simulink model "sampleModel1527"  (R2023a)
settings: Solver=VariableStepAuto  StartTime=0.0  StopTime=10.0  RelTol=1e-3
libraries: hdlsllib x3, simulink x3
settings Model: Creator=user1  LastModifiedBy=user1

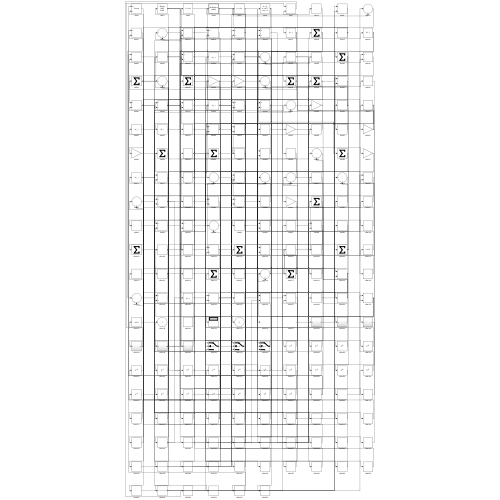
[thumbnail: Simulink's stored preview of the top-level diagram]
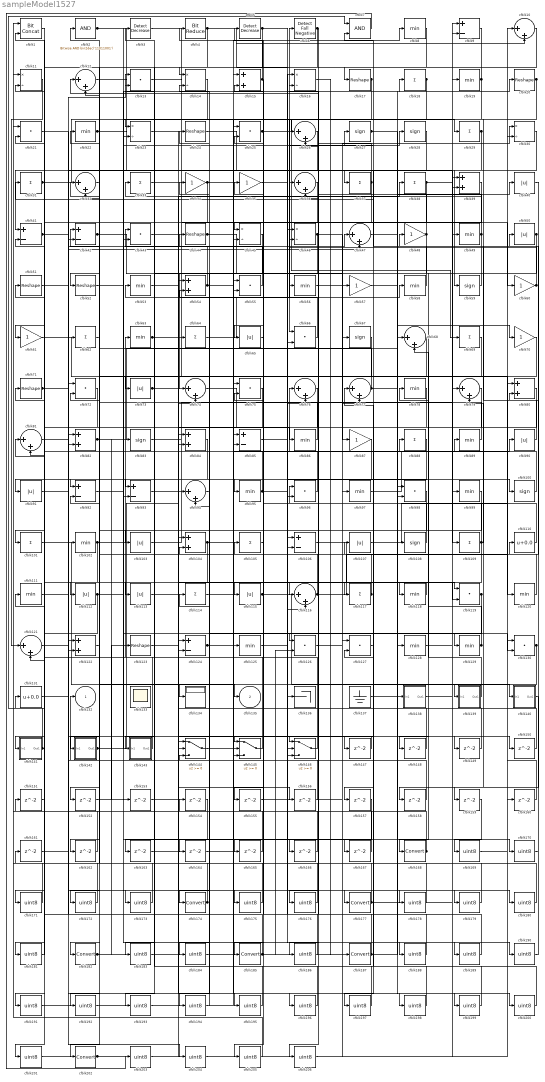
== system sampleModel1527 ==
  cfblk1 : hdlsllib/Logic and Bit Operations/Bit Concat  numInputs=2
  cfblk{10,12,26,32,36,47,68,74,76..77,79,81,94,116,121} (15 alike) : Sum  Inputs=|++
  cfblk{27..28,59,67,83,100,108} (7 alike) : Signum
  cfblk{18,29,31,33,37..38,62,64,69,88,101,105,109,114,117} (15 alike) : Sum  Inputs=+
  cfblk{8,19,22,49,53,56,58,63,78,86,89,95,97,99,102,111,118,120,125,128..129} (21 alike) : MinMax
  cfblk{40,50,65,73,90..91,103,107,112..113,115} (11 alike) : Abs  SaturateOnIntegerOverflow=off
  cfblk{15,39,54,80,82,84,104,122} (8 alike) : Sum
  cfblk{9,41..42,85,92..93,106,124} (8 alike) : Sum  Inputs=+-
  cfblk{11,14,16,23,30,45..46} (7 alike) : Product  Inputs=*/  RndMeth=Zero  SaturateOnIntegerOverflow=on
  cfblk110 : Bias  Bias=0.0  SaturateOnIntegerOverflow=off
  cfblk{13,21,25,43,55,66,72,75,96,98,119,126..127,130} (14 alike) : DotProduct  OutDataTypeStr=Inherit: Inherit via internal rule
  cfblk{17,20,24,44,51..52,71,123} (8 alike) : Reshape
  cfblk131 : Bias  Bias=0.0  SaturateOnIntegerOverflow=off
  cfblk133 : Scope
      settings: Floating=on
  cfblk134 : Display
  cfblk136 : Terminator
  cfblk137 : Ground
  cfblk138 : Subsystem
      settings: LibrarySourceBlock=|
      | hdlsllib/Ports &
      | Subsystems/Subsystem
  cfblk139 : Subsystem
      settings: LibrarySourceBlock=|
      | hdlsllib/Ports &
      | Subsystems/Subsystem
  cfblk140 : Subsystem
      settings: LibrarySourceBlock=|
      | hdlsllib/Ports &
      | Subsystems/Subsystem
  cfblk141 : Subsystem
      settings: LibrarySourceBlock=|
      | hdlsllib/Ports &
      | Subsystems/Subsystem
  cfblk142 : Subsystem
      settings: LibrarySourceBlock=|
      | hdlsllib/Ports &
      | Subsystems/Subsystem
  cfblk143 : Subsystem
      settings: LibrarySourceBlock=|
      | hdlsllib/Ports &
      | Subsystems/Subsystem
  cfblk144 : Switch  SaturateOnIntegerOverflow=off  InputSameDT=off
  cfblk145 : Switch  SaturateOnIntegerOverflow=off  InputSameDT=off
  cfblk146 : Switch  SaturateOnIntegerOverflow=off  InputSameDT=off
  cfblk{147..167} (21 alike) : Delay  SampleTime=1
  cfblk{168,174,177,182,185,187,202} (7 alike) : DataTypeConversion  SaturateOnIntegerOverflow=off  RndMeth=Floor
  cfblk{169..173,175..176,178..181,183..184,186,188..201,203..206} (32 alike) : DataTypeConversion  OutDataTypeStr=uint8  SaturateOnIntegerOverflow=off  RndMeth=Floor
  cfblk2 : simulink/Logic and Bit Operations/Bitwise Operator  logicop=AND  UseBitMask=on  BitMask=bin2dec('11011001')  BitMaskRealWorld=Stored Integer
      settings: LibrarySourceBlock=|
      | hdlsllib/Logic and Bit
      | Operations/Bitwise
      | Operator
  cfblk3 : simulink/Logic and Bit Operations/Detect Decrease  vinit=0.0  OutDataTypeStr=boolean
      settings: LibrarySourceBlock=|
      | hdlsllib/Logic and Bit
      | Operations/Detect
      | Decrease
  cfblk{34..35,48,57,60..61,70,87} (8 alike) : Gain
  cfblk4 : hdlsllib/Logic and Bit Operations/Bit Reduce  mode=AND
  cfblk5 : simulink/Logic and Bit Operations/Detect Decrease  vinit=0.0  OutDataTypeStr=boolean
      settings: LibrarySourceBlock=|
      | hdlsllib/Logic and Bit
      | Operations/Detect
      | Decrease
  cfblk6 : hdlsllib/Logic and Bit Operations/Detect Fall Negative  vinit=0  OutDataTypeStr=boolean
  cfblk7 : Logic  AllPortsSameDT=off  OutDataTypeStr=boolean
  cfblk132 : Outport  VectorParamsAs1DForOutWhenUnconnected=off
  cfblk135 : Outport  Port=2  VectorParamsAs1DForOutWhenUnconnected=off
  wires:
  cfblk29/1 -> cfblk59/1, cfblk36/1
  cfblk34/1 -> cfblk42/2, cfblk117/1, cfblk201/1
  cfblk145/1 -> cfblk63/1
  cfblk20/1 -> cfblk145/2, cfblk159/1
  cfblk37/1 -> cfblk12/1, cfblk45/2
  cfblk43/1 -> cfblk58/1
  cfblk106/1 -> cfblk119/1
  cfblk22/1 -> cfblk84/2, cfblk178/1
  cfblk65/1 -> cfblk132/1
  cfblk31/1 -> cfblk69/1, cfblk37/1
  cfblk119/1 -> cfblk155/1, cfblk194/1
  cfblk110/1 -> cfblk96/1
  cfblk48/1 -> cfblk74/1, cfblk7/2
  cfblk77/1 -> cfblk12/2, cfblk20/1
  cfblk17/1 -> cfblk66/1, cfblk176/1
  cfblk64/1 -> cfblk6/1
  cfblk103/1 -> cfblk9/1
  cfblk90/1 -> cfblk48/1
  cfblk39/1 -> cfblk202/1
  cfblk3/1 -> cfblk45/1
  cfblk88/1 -> cfblk134/1
  cfblk52/1 -> cfblk28/1
  cfblk9/1 -> cfblk52/1
  cfblk11/1 -> cfblk121/1
  cfblk13/1 -> cfblk120/1
  cfblk100/1 -> cfblk51/1
  cfblk114/1 -> cfblk177/1
  cfblk54/1 -> cfblk43/1, cfblk118/1
  cfblk27/1 -> cfblk70/1, cfblk140/1(In1)
  cfblk28/1 -> cfblk93/1
  cfblk124/1 -> cfblk15/1, cfblk90/1
  cfblk113/1 -> cfblk146/1
  cfblk63/1 -> cfblk94/1, cfblk116/1
  cfblk130/1 -> cfblk162/1, cfblk163/1, cfblk186/1
  cfblk68/1 -> cfblk96/2
  cfblk128/1 -> cfblk49/1
  cfblk142/1(Out1) -> cfblk38/1, cfblk18/1
  cfblk74/1 -> cfblk106/1
  cfblk97/1 -> cfblk89/1
  cfblk19/1 -> cfblk17/1, cfblk43/2
  cfblk56/1 -> cfblk30/1
  cfblk101/1 -> cfblk135/1
  cfblk104/1 -> cfblk8/1, cfblk142/1(In1)
  cfblk59/1 -> cfblk54/1
  cfblk102/1 -> cfblk64/1, cfblk112/1
  cfblk14/1 -> cfblk93/2
  cfblk25/1 -> cfblk29/1, cfblk100/1
  cfblk117/1 -> cfblk107/1, cfblk36/2
  cfblk40/1 -> cfblk110/1
  cfblk93/1 -> cfblk56/1
  cfblk6/1 -> cfblk143/1(In1), cfblk166/1
  cfblk120/1 -> cfblk42/1
  cfblk139/1(Out1) -> cfblk88/1
  cfblk50/1 -> cfblk55/2, cfblk148/1
  cfblk44/1 -> cfblk87/1, cfblk130/2, cfblk188/1
  cfblk92/1 -> cfblk124/2
  cfblk137/1 -> cfblk68/1
  cfblk138/1(Out1) -> cfblk19/1
  cfblk108/1 -> cfblk35/1
  cfblk26/1 -> cfblk41/1
  cfblk75/1 -> cfblk174/1
  cfblk109/1 -> cfblk121/2, cfblk79/2, cfblk5/1
  cfblk42/1 -> cfblk27/1, cfblk146/3, cfblk76/2
  cfblk24/1 -> cfblk109/1
  cfblk146/1 -> cfblk41/2
  cfblk141/1(Out1) -> cfblk7/1, cfblk11/2
  cfblk105/1 -> cfblk185/1
  cfblk58/1 -> cfblk26/1
  cfblk82/1 -> cfblk40/1, cfblk153/1
  cfblk33/1 -> cfblk60/1
  cfblk49/1 -> cfblk33/1, cfblk126/1, cfblk26/2
  cfblk96/1 -> cfblk76/1
  cfblk45/1 -> cfblk103/1
  cfblk51/1 -> cfblk82/2
  cfblk107/1 -> cfblk10/1
  cfblk94/1 -> cfblk34/1
  cfblk62/1 -> cfblk92/1
  cfblk35/1 -> cfblk136/1
  cfblk126/1 -> cfblk97/1
  cfblk21/1 -> cfblk102/1
  cfblk116/1 -> cfblk30/2, cfblk14/2
  cfblk15/1 -> cfblk4/1, cfblk95/1
  cfblk38/1 -> cfblk9/2, cfblk61/1
  cfblk1/1 -> cfblk91/1
  cfblk2/1 -> cfblk108/1, cfblk145/1, cfblk189/1
  cfblk118/1 -> cfblk113/1
  cfblk83/1 -> cfblk66/2
  cfblk112/1 -> cfblk141/1(In1), cfblk167/1
  cfblk10/1 -> cfblk101/1
  cfblk4/1 -> cfblk14/1, cfblk10/2, cfblk116/2
  cfblk98/1 -> cfblk182/1
  cfblk5/1 -> cfblk119/2, cfblk23/2
  cfblk18/1 -> cfblk23/1, cfblk206/1
  cfblk86/1 -> cfblk54/2
  cfblk95/1 -> cfblk2/1, cfblk115/1, cfblk170/1
  cfblk143/1(Out1) -> cfblk71/1
  cfblk46/1 -> cfblk67/1, cfblk184/1
  cfblk125/1 -> cfblk46/1
  cfblk115/1 -> cfblk139/1(In1), cfblk165/1
  cfblk78/1 -> cfblk122/2
  cfblk73/1 -> cfblk3/1, cfblk129/1
  cfblk12/1 -> cfblk125/1
  cfblk61/1 -> cfblk106/2
  cfblk122/1 -> cfblk32/1
  cfblk131/1 -> cfblk13/1
  cfblk41/1 -> cfblk150/1, cfblk175/1
  cfblk89/1 -> cfblk22/1
  cfblk55/1 -> cfblk24/1
  cfblk76/1 -> cfblk146/2
  cfblk36/1 -> cfblk65/1
  cfblk66/1 -> cfblk13/2
  cfblk121/1 -> cfblk47/1
  cfblk16/1 -> cfblk187/1
  cfblk8/1 -> cfblk73/1
  cfblk60/1 -> cfblk46/2, cfblk31/1
  cfblk23/1 -> cfblk86/1
  cfblk80/1 -> cfblk168/1
  cfblk129/1 -> cfblk78/1, cfblk68/2
  cfblk71/1 -> cfblk62/1, cfblk47/2
  cfblk30/1 -> cfblk147/1
  cfblk147/1 -> cfblk144/2
  cfblk148/1 -> cfblk124/1
  cfblk47/1 -> cfblk149/1
  cfblk149/1 -> cfblk15/2
  cfblk150/1 -> cfblk104/1
  cfblk151/1 -> cfblk21/2
  cfblk84/1 -> cfblk152/1
  cfblk155/1 -> cfblk77/2
  cfblk123/1 -> cfblk156/1
  cfblk156/1 -> cfblk92/2
  cfblk70/1 -> cfblk157/1
  cfblk140/1(Out1) -> cfblk158/1
  cfblk158/1 -> cfblk122/1
  cfblk160/1 -> cfblk130/1
  cfblk162/1 -> cfblk1/1
  cfblk163/1 -> cfblk145/3
  cfblk69/1 -> cfblk164/1
  cfblk164/1 -> cfblk94/2
  cfblk165/1 -> cfblk1/2
  cfblk166/1 -> cfblk144/3
  cfblk167/1 -> cfblk32/2
  cfblk168/1 -> cfblk83/1, cfblk77/1
  cfblk159/1 -> cfblk169/1
  cfblk169/1 -> cfblk80/1
  cfblk170/1 -> cfblk80/2
  cfblk72/1 -> cfblk171/1
  cfblk171/1 -> cfblk21/1
  cfblk32/1 -> cfblk172/1
  cfblk172/1 -> cfblk72/1
  cfblk161/1 -> cfblk173/1
  cfblk173/1 -> cfblk72/2
  cfblk174/1 -> cfblk151/1, cfblk84/1
  cfblk175/1 -> cfblk75/1
  cfblk176/1 -> cfblk75/2
  cfblk177/1 -> cfblk131/1, cfblk79/1, cfblk111/1
  cfblk178/1 -> cfblk114/1
  cfblk81/1 -> cfblk179/1
  cfblk179/1 -> cfblk25/1
  cfblk152/1 -> cfblk180/1
  cfblk180/1 -> cfblk81/1
  cfblk79/1 -> cfblk181/1
  cfblk181/1 -> cfblk81/2
  cfblk182/1 -> cfblk138/1(In1), cfblk123/1
  cfblk157/1 -> cfblk183/1
  cfblk183/1 -> cfblk98/1
  cfblk184/1 -> cfblk98/2
  cfblk185/1 -> cfblk161/1, cfblk126/2, cfblk82/1
  cfblk186/1 -> cfblk105/1
  cfblk187/1 -> cfblk128/1, cfblk25/2
  cfblk188/1 -> cfblk16/1
  cfblk189/1 -> cfblk16/2
  cfblk85/1 -> cfblk190/1
  cfblk190/1 -> cfblk50/1
  cfblk87/1 -> cfblk191/1
  cfblk191/1 -> cfblk85/1
  cfblk67/1 -> cfblk192/1
  cfblk192/1 -> cfblk85/2
  cfblk154/1 -> cfblk193/1
  cfblk193/1 -> cfblk55/1
  cfblk194/1 -> cfblk154/1
  cfblk53/1 -> cfblk195/1
  cfblk195/1 -> cfblk144/1
  cfblk91/1 -> cfblk196/1
  cfblk196/1 -> cfblk53/1
  cfblk127/1 -> cfblk197/1
  cfblk197/1 -> cfblk104/2
  cfblk144/1 -> cfblk198/1
  cfblk198/1 -> cfblk127/1
  cfblk153/1 -> cfblk199/1
  cfblk199/1 -> cfblk127/2
  cfblk57/1 -> cfblk200/1
  cfblk200/1 -> cfblk44/1
  cfblk201/1 -> cfblk57/1
  cfblk202/1 -> cfblk160/1, cfblk74/2
  cfblk7/1 -> cfblk203/1
  cfblk203/1 -> cfblk39/1
  cfblk111/1 -> cfblk204/1
  cfblk204/1 -> cfblk39/2
  cfblk99/1 -> cfblk205/1
  cfblk205/1 -> cfblk11/1
  cfblk206/1 -> cfblk99/1

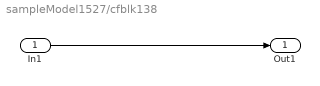
== system sampleModel1527/cfblk138 ==
  In1 : Inport
  Out1 : Outport
  wires:
  In1/1 -> Out1/1

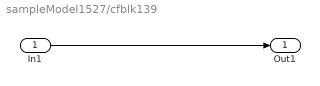
== system sampleModel1527/cfblk139 ==
  In1 : Inport
  Out1 : Outport
  wires:
  In1/1 -> Out1/1

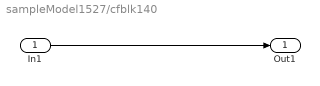
== system sampleModel1527/cfblk140 ==
  In1 : Inport
  Out1 : Outport
  wires:
  In1/1 -> Out1/1

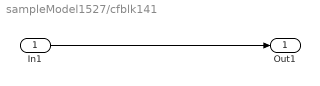
== system sampleModel1527/cfblk141 ==
  In1 : Inport
  Out1 : Outport
  wires:
  In1/1 -> Out1/1

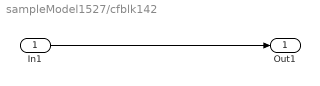
== system sampleModel1527/cfblk142 ==
  In1 : Inport
  Out1 : Outport
  wires:
  In1/1 -> Out1/1

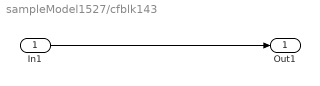
== system sampleModel1527/cfblk143 ==
  In1 : Inport
  Out1 : Outport
  wires:
  In1/1 -> Out1/1
